simulink model "Mass-Spring-Damper-NonlinearModel_simulink"  (R2019b)
settings: Solver=VariableStepAuto  StartTime=0.0  StopTime=10.0  RelTol=1e-3
settings Model: Creator=Bekircan Keceoglu  LastModifiedBy=Bekircan Keceoglu

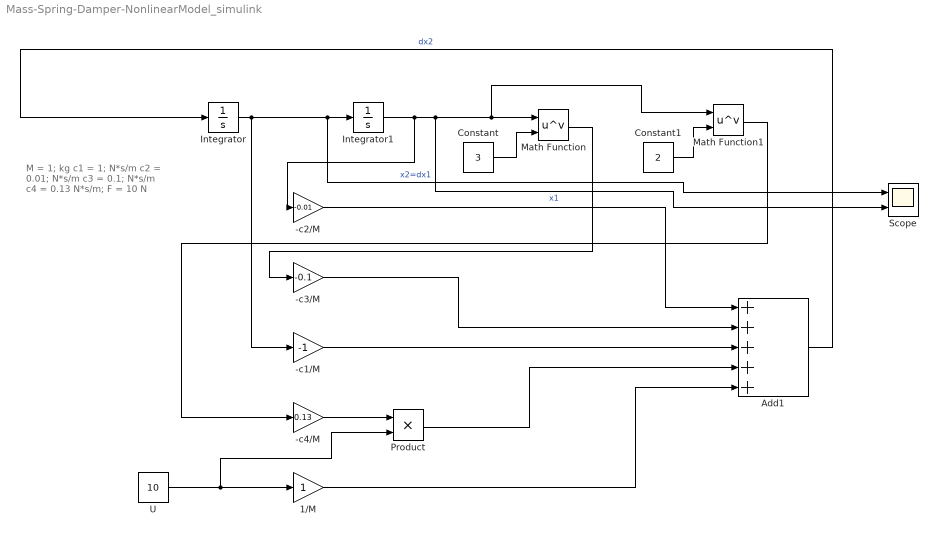
== system Mass-Spring-Damper-NonlinearModel_simulink ==
  note: M  = 1; kg
      | c1 = 1;  N*s/m
      | c2 = 0.01; N*s/m
      | c3 = 0.1; N*s/m
      | c4 = 0.13 N*s/m;
      | F  = 10 N
  -c1/M : Gain  Gain=-1
  -c2/M : Gain  Gain=-0.01
  -c3/M : Gain  Gain=-0.1
  -c4/M : Gain  Gain=0.13
  1/M : Gain
  Add1 : Sum  Inputs=+++++
  Constant : Constant  Value=3
  Constant1 : Constant  Value=2
  Integrator : Integrator
  Integrator1 : Integrator
  Math Function : Math  Operator=pow  SignedPower=off  SaturateOnIntegerOverflow=on
  Math Function1 : Math  Operator=pow  SignedPower=off  SaturateOnIntegerOverflow=on
  Product : Product
  Scope : Scope  NumInputPorts=2
  U : Constant  Value=10
  wires:
  Integrator/1 -> -c1/M/1, Scope/1, Integrator1/1  "x2=dx1"
  Integrator1/1 -> -c2/M/1, Scope/2, Math Function1/1, Math Function/1  "x1"
  Add1/1 -> Integrator/1  "dx2"
  Constant/1 -> Math Function/2
  Constant1/1 -> Math Function1/2
  Math Function/1 -> -c3/M/1
  -c2/M/1 -> Add1/1
  -c3/M/1 -> Add1/2
  -c1/M/1 -> Add1/3
  U/1 -> Product/2, 1/M/1
  1/M/1 -> Add1/5
  Math Function1/1 -> -c4/M/1
  -c4/M/1 -> Product/1
  Product/1 -> Add1/4
